simulink model "modelo_global_NL"  (R2020a)
settings: Solver=VariableStepAuto  StartTime=0.0  StopTime=10.0  RelTol=1e-3
model workspace: external: MATLAB File D:\Ferran\Facultad\UNCuyo\Meca\Automática y Máquinas Eléctricas\Proyecto final\matlab2\parametros_y_especs\parametros_y_especif.m (data not in the file)
undefined symbols (not defined in the file): alpha_Cu, beq, Cts, Jeq, L_ls, lambda_m, Ld, Lq, magnitude, Pp, r, Rref, Rts_amb, Tref
settings Model: Creator=Ferran  LastModifiedBy=Ferran

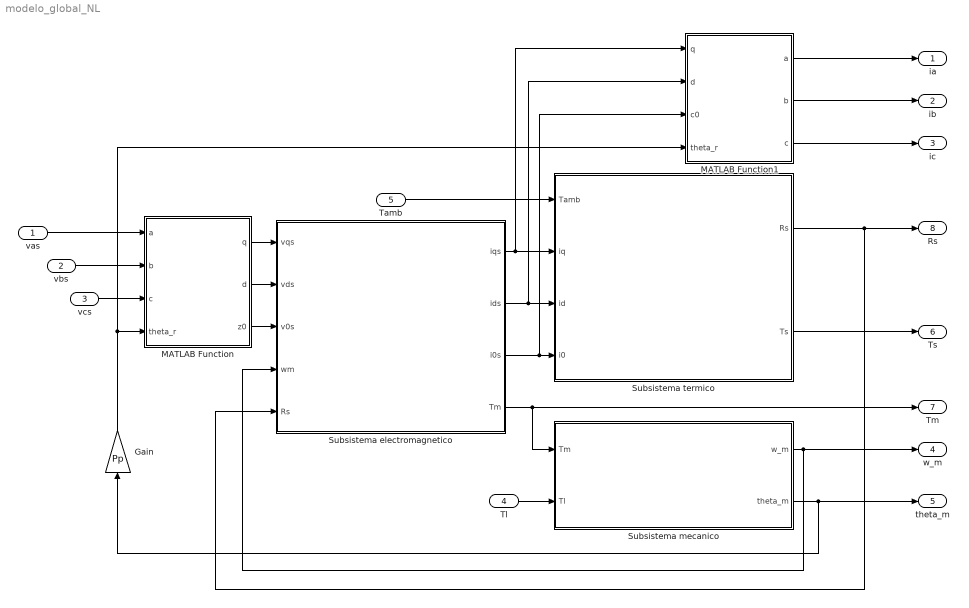
== system modelo_global_NL ==
  vas : Inport
  vbs : Inport  Port=2
  vcs : Inport  Port=3
  Tl : Inport  Port=4
  Tamb : Inport  Port=5
  Gain : Gain  Gain=Pp
  MATLAB Function : MATLAB Function  TreatAsAtomicUnit=on
  MATLAB Function1 : MATLAB Function  TreatAsAtomicUnit=on
  Subsistema electromagnetico : Subsystem
  Subsistema mecanico : Subsystem
  Subsistema termico : Subsystem
  ia : Outport
  ib : Outport  Port=2
  ic : Outport  Port=3
  w_m : Outport  Port=4
  theta_m : Outport  Port=5
  Ts : Outport  Port=6
  Tm : Outport  Port=7
  Rs : Outport  Port=8
  wires:
  vas/1 -> MATLAB Function/1(a)
  vbs/1 -> MATLAB Function/2(b)
  vcs/1 -> MATLAB Function/3(c)
  MATLAB Function/1(q) -> Subsistema electromagnetico/1(vqs)
  MATLAB Function/2(d) -> Subsistema electromagnetico/2(vds)
  MATLAB Function/3(z0) -> Subsistema electromagnetico/3(v0s)
  Subsistema electromagnetico/1(iqs) -> Subsistema termico/2(iq), MATLAB Function1/1(q)
  Subsistema electromagnetico/2(ids) -> Subsistema termico/3(id), MATLAB Function1/2(d)
  Subsistema electromagnetico/3(i0s) -> Subsistema termico/4(i0), MATLAB Function1/3(c0)
  Tl/1 -> Subsistema mecanico/2(Tl)
  Subsistema electromagnetico/4(Tm) -> Tm/1, Subsistema mecanico/1(Tm)
  Tamb/1 -> Subsistema termico/1(Tamb)
  MATLAB Function1/1(a) -> ia/1
  MATLAB Function1/2(b) -> ib/1
  MATLAB Function1/3(c) -> ic/1
  Subsistema termico/1(Rs) -> Subsistema electromagnetico/5(Rs), Rs/1
  Subsistema termico/2(Ts) -> Ts/1
  Subsistema mecanico/1(w_m) -> Subsistema electromagnetico/4(wm), w_m/1
  Subsistema mecanico/2(theta_m) -> theta_m/1, Gain/1
  Gain/1 -> MATLAB Function/4(theta_r), MATLAB Function1/4(theta_r)

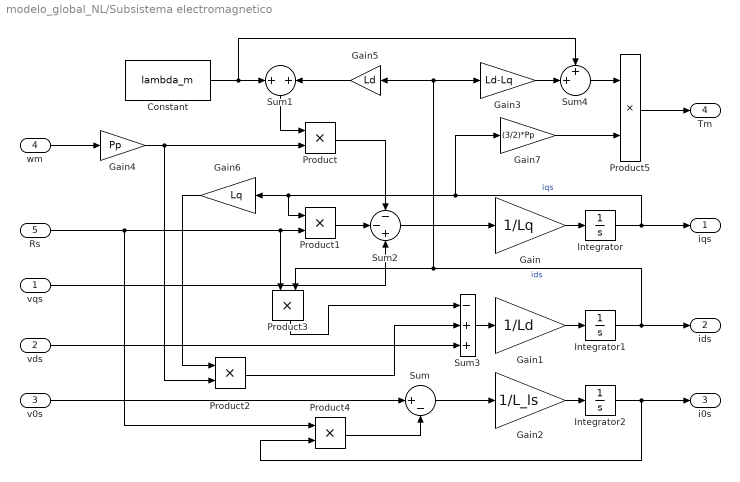
== system modelo_global_NL/Subsistema electromagnetico ==
  vqs : Inport
  vds : Inport  Port=2
  v0s : Inport  Port=3
  wm : Inport  Port=4
  Rs : Inport  Port=5
  Constant : Constant  Value=lambda_m
  Gain : Gain  Gain=1/Lq
  Gain1 : Gain  Gain=1/Ld
  Gain2 : Gain  Gain=1/L_ls
  Gain3 : Gain  Gain=Ld-Lq
  Gain4 : Gain  Gain=Pp
  Gain5 : Gain  Gain=Ld
  Gain6 : Gain  Gain=Lq
  Gain7 : Gain  Gain=(3/2)*Pp
  Integrator : Integrator
  Integrator1 : Integrator
  Integrator2 : Integrator
  Product{,1..5} (6 alike) : Product
  Sum : Sum  Inputs=|+-
  Sum1 : Sum  Inputs=+|+
  Sum2 : Sum  Inputs=--+
  Sum3 : Sum  Inputs=-++
  Sum4 : Sum  Inputs=++|
  iqs : Outport
  ids : Outport  Port=2
  i0s : Outport  Port=3
  Tm : Outport  Port=4
  wires:
  Constant/1 -> Sum1/1, Sum4/1
  Product1/1 -> Sum2/2
  Rs/1 -> Product1/2, Product3/1, Product4/1
  Integrator/1 -> iqs/1, Gain7/1, Gain6/1, Product1/1  "iqs"
  Gain3/1 -> Sum4/2
  Sum/1 -> Gain2/1
  Sum2/1 -> Gain/1
  vqs/1 -> Sum2/3
  Product3/1 -> Sum3/1
  Product4/1 -> Sum/2
  vds/1 -> Sum3/3
  Sum3/1 -> Gain1/1
  Gain6/1 -> Product2/1
  Integrator1/1 -> ids/1, Product3/2, Gain5/1, Gain3/1  "ids"
  Product2/1 -> Sum3/2
  Integrator2/1 -> i0s/1, Product4/2
  wm/1 -> Gain4/1
  Sum1/1 -> Product/1
  Gain5/1 -> Sum1/2
  Product/1 -> Sum2/1
  Gain/1 -> Integrator/1
  v0s/1 -> Sum/1
  Gain2/1 -> Integrator2/1
  Gain1/1 -> Integrator1/1
  Gain7/1 -> Product5/2
  Product5/1 -> Tm/1
  Gain4/1 -> Product/2, Product2/2
  Sum4/1 -> Product5/1

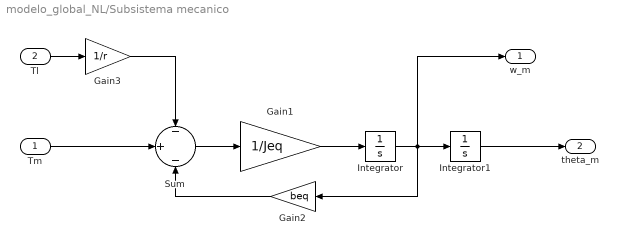
== system modelo_global_NL/Subsistema mecanico ==
  Tm : Inport
  Tl : Inport  Port=2
  Gain1 : Gain  Gain=1/Jeq
  Gain2 : Gain  Gain=beq
  Gain3 : Gain  Gain=1/r
  Integrator : Integrator
  Integrator1 : Integrator
  Sum : Sum  Inputs=-|+|-
  w_m : Outport
  theta_m : Outport  Port=2
  wires:
  Tm/1 -> Sum/2
  Gain3/1 -> Sum/1
  Integrator/1 -> w_m/1, Gain2/1, Integrator1/1
  Integrator1/1 -> theta_m/1
  Gain2/1 -> Sum/3
  Sum/1 -> Gain1/1
  Tl/1 -> Gain3/1
  Gain1/1 -> Integrator/1

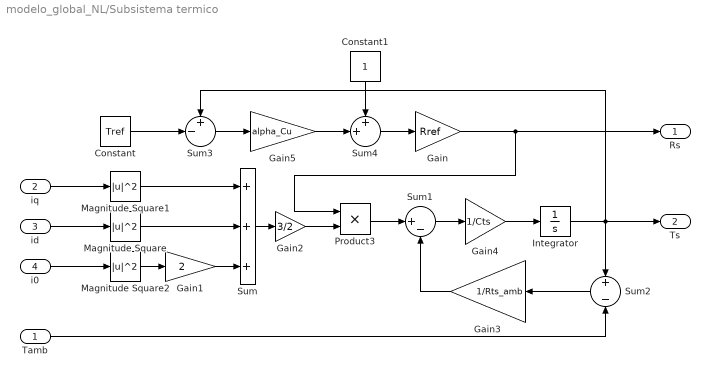
== system modelo_global_NL/Subsistema termico ==
  Tamb : Inport
  iq : Inport  Port=2
  id : Inport  Port=3
  i0 : Inport  Port=4
  Constant : Constant  Value=Tref
  Constant1 : Constant
  Gain : Gain  Gain=Rref
  Gain1 : Gain  Gain=2
  Gain2 : Gain  Gain=3/2
  Gain3 : Gain  Gain=1/Rts_amb
  Gain4 : Gain  Gain=1/Cts
  Gain5 : Gain  Gain=alpha_Cu
  Integrator : Integrator  InitialCondition=40
  Magnitude Square : Math  Operator=magnitude^2  SignedPower=on  RndMeth=Zero  SaturateOnIntegerOverflow=on
  Magnitude Square1 : Math  Operator=magnitude^2  SignedPower=on  RndMeth=Zero  SaturateOnIntegerOverflow=on
  Magnitude Square2 : Math  Operator=magnitude^2  SignedPower=on  RndMeth=Zero  SaturateOnIntegerOverflow=on
  Product3 : Product
  Sum : Sum  Inputs=+++
  Sum1 : Sum  Inputs=|+-
  Sum2 : Sum  Inputs=+-
  Sum3 : Sum  Inputs=+-|
  Sum4 : Sum  Inputs=++|
  Rs : Outport
  Ts : Outport  Port=2
  wires:
  Magnitude Square1/1 -> Sum/1
  id/1 -> Magnitude Square/1
  Sum2/1 -> Gain3/1
  i0/1 -> Magnitude Square2/1
  Gain4/1 -> Integrator/1
  iq/1 -> Magnitude Square1/1
  Sum/1 -> Gain2/1
  Gain3/1 -> Sum1/2
  Gain2/1 -> Product3/2
  Sum1/1 -> Gain4/1
  Gain5/1 -> Sum4/2
  Product3/1 -> Sum1/1
  Tamb/1 -> Sum2/2
  Gain/1 -> Rs/1, Product3/1
  Sum3/1 -> Gain5/1
  Sum4/1 -> Gain/1
  Magnitude Square/1 -> Sum/2
  Magnitude Square2/1 -> Gain1/1
  Gain1/1 -> Sum/3
  Constant1/1 -> Sum4/1
  Integrator/1 -> Ts/1, Sum3/1, Sum2/1
  Constant/1 -> Sum3/2

== matlab function modelo_global_NL/MATLAB Function1 ==
  data: q input; a output; d input; c0 input; theta_r input; b output; c output
function [a,b,c] = TPark_inversa(q,d,c0,theta_r)
    fqd0 = [q;d;c0];
    T = [cos(theta_r)               sin(theta_r)            1;
        cos(theta_r - (2*pi)/3)    sin(theta_r - (2*pi)/3) 1;
        cos(theta_r + (2*pi)/3)    sin(theta_r + (2*pi)/3) 1];
    
    fabc = T*fqd0;
    
    a = fabc(1);
    b = fabc(2);
    c = fabc(3);
end

== matlab function modelo_global_NL/MATLAB Function ==
  data: a input; q output; b input; c input; theta_r input; d output; z0 output
function [q,d,z0] = TPark_directa(a,b,c,theta_r)
    fabc = [a;b;c];
    T = (2/3) * ...
        [ cos(theta_r) cos(theta_r - (2*pi)/3) cos(theta_r + (2*pi)/3);
        sin(theta_r) sin(theta_r - (2*pi)/3) sin(theta_r + (2*pi)/3);
        1/2                   1/2                  1/2];
  
  fqd0 = T*fabc;
  q = fqd0(1);
  d = fqd0(2);
  z0 = fqd0(3);
end
